simulink model "PRegler"  (R2025b)
settings: Solver=VariableStepAuto  StartTime=0  StopTime=run_time  FixedStep=1e-5  MaxStep=1e-5  RelTol=1e-3
values from neighbouring files (symbols this model uses):
  K = 10    [PID_Regler.m]
settings Model: Creator=ruth  LastModifiedBy=ruth

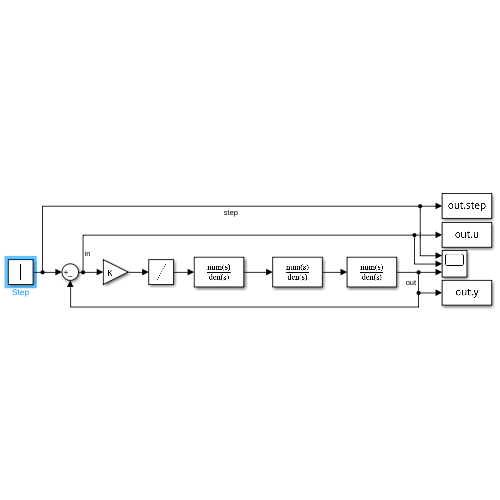
[thumbnail: Simulink's stored preview of the top-level diagram]
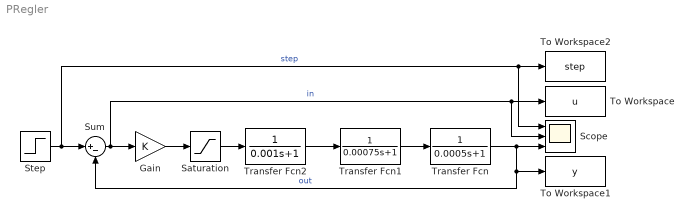
== system PRegler ==
  Gain : Gain  Gain=K
  Saturation : Saturate  UpperLimit=12  LowerLimit=-12
  Scope : Scope  NumInputPorts=3
      settings: ActiveDisplayYMinimum=-1.9754584907399237  ActiveDisplayYMaximum=5.975458490739924
  Step : Step  Time=0  After=4  SampleTime=0
  Sum : Sum  Inputs=|+-
  To Workspace : ToWorkspace  VariableName=u  SaveFormat=Timeseries  SampleTime=-1
  To Workspace1 : ToWorkspace  VariableName=y  SaveFormat=Timeseries  SampleTime=-1
  To Workspace2 : ToWorkspace  VariableName=step  SaveFormat=Timeseries  SampleTime=-1
  Transfer Fcn : TransferFcn  Denominator=[0.0005 1]
  Transfer Fcn1 : TransferFcn  Denominator=[0.00075 1]
  Transfer Fcn2 : TransferFcn  Denominator=[0.001 1]
  wires:
  Transfer Fcn/1 -> Sum/2, To Workspace1/1, Scope/3  "out"
  Step/1 -> Scope/1, To Workspace2/1, Sum/1  "step"
  Sum/1 -> Scope/2, To Workspace/1, Gain/1  "in"
  Transfer Fcn1/1 -> Transfer Fcn/1
  Transfer Fcn2/1 -> Transfer Fcn1/1
  Gain/1 -> Saturation/1
  Saturation/1 -> Transfer Fcn2/1
